simulink model "TV2016_CAN"  (Simulink 8.5)
settings: Solver=ode1  StartTime=0.0  StopTime=inf  FixedStep=0.001  RelTol=1e-3
PreLoadFcn:
  | FSE_Parameters
values from neighbouring files (symbols this model uses):
  car_params = Simulink_Car_params    [TV2016_parameters.m]
  i_Diff = 15.47    [TV2016_parameters.m]
  Kp = 1    [TV2016_parameters.m]
  settings = Simulink_Settings    [TV2016_parameters.m]
  SpdC_BCC = 0    [TV2016_parameters.m]
  Speed_Neg_sat = -21    [TV2016_parameters.m]
  Speed_Pos_sat = 21    [TV2016_parameters.m]
  Tn_n = 0    [TV2016_parameters.m]
  Use_Joystick = 1    [TV2016_parameters.m]
undefined symbols (not defined in the file or in its folder): canChannel
libraries: CarMaker4SL x139, simulink x18, canmsglib x10, simulink_extras x7, canlib x5, sldrtlib x1
(part 2 of 4)

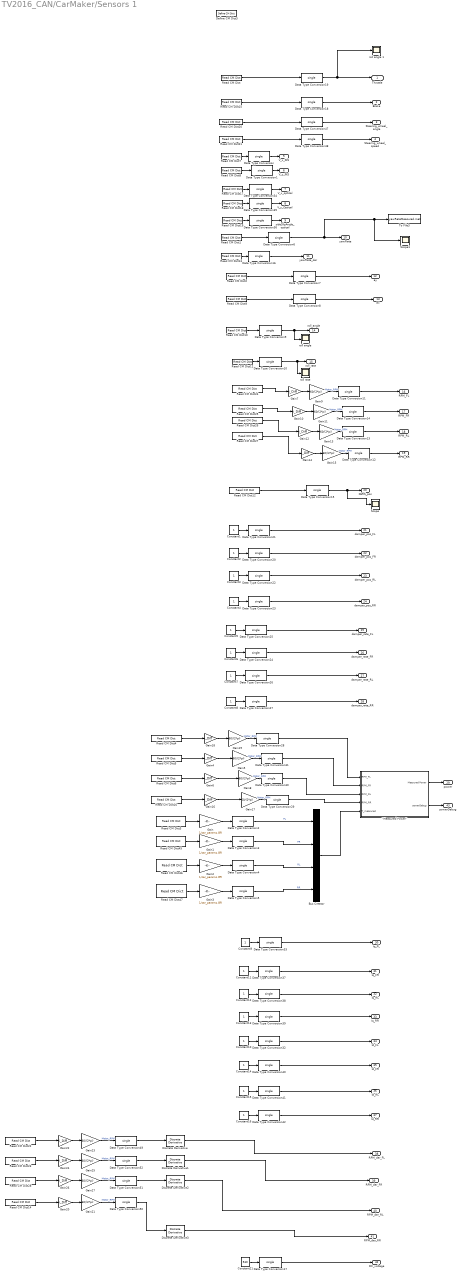
== system TV2016_CAN/CarMaker/Sensors 1 ==
  "\"Measured Power\"" : Subsystem
  Bus Creator : BusCreator  OutDataTypeStr=Bus: T_meas
      settings: InheritFromInputs=off
  Constant{1..16} (16 alike) : Constant
  Constant21 : Constant  Value=530
  Data Type Conversion{,1..42,47..52} (49 alike) : DataTypeConversion  OutDataTypeStr=single
  Define CM Dict3 : CarMaker4SL/Define CM Dict  xname=KERS_pos  xmono=off  xtype=Double  xdvaplace=None  xnstates=0  xfirststate=0  xinitial=0
  Discrete Derivative{,1..3} (4 alike) : simulink/Discrete/Discrete Derivative  gainval=1.0  ICPrevScaledInput=0.0  InputProcessing=Inherited  OutMin=[]  OutMax=[]  OutDataType=fixdt(1, 16)  OutScaling=2^-10  DoSatur=off
  Gain{,1..3} (4 alike) : Gain  Gain=1/car_params.GR
  Gain{4,6..7,10,12,14,16,18,20,22,24,26} (12 alike) : Gain  Gain=i_Diff
  Gain{5,8..9,11,13,15,17,19,21,23,25,27} (12 alike) : Gain  Gain=60/(2*pi)
  Read CM Dict : CarMaker4SL/Read CM Dict  xname=VC.Gas  xsync=off
  Read CM Dict1 : CarMaker4SL/Read CM Dict  xname=Vhcl.YawRate  xsync=off
  Read CM Dict10 : CarMaker4SL/Read CM Dict  xname=Vhcl.Roll  xsync=off
  Read CM Dict11 : CarMaker4SL/Read CM Dict  xname=Vhcl.RollVel  xsync=off
  Read CM Dict12 : CarMaker4SL/Read CM Dict  xname=KERS_pos  xsync=off
  Read CM Dict13 : CarMaker4SL/Read CM Dict  xname=Vhcl.YawAcc  xsync=off
  Read CM Dict14 : CarMaker4SL/Read CM Dict  xname=Car.WheelSpd_RR  xsync=off
  Read CM Dict15 : CarMaker4SL/Read CM Dict  xname=VC.Brake  xsync=off
  Read CM Dict16 : CarMaker4SL/Read CM Dict  xname=Car.WheelSpd_RR  xsync=off
  Read CM Dict17 : CarMaker4SL/Read CM Dict  xname=Car.vx  xsync=off
  Read CM Dict18 : CarMaker4SL/Read CM Dict  xname=Car.vy  xsync=off
  Read CM Dict19 : CarMaker4SL/Read CM Dict  xname=Car.SideSlipAngle  xsync=off
  Read CM Dict2 : CarMaker4SL/Read CM Dict  xname=Car.ay  xsync=off
  Read CM Dict20 : CarMaker4SL/Read CM Dict  xname=Vhcl.Steer.Ang  xsync=off
  Read CM Dict21 : CarMaker4SL/Read CM Dict  xname=Vhcl.Steer.Vel  xsync=off
  Read CM Dict22 : CarMaker4SL/Read CM Dict  xname=Car.WheelSpd_FL  xsync=off
  Read CM Dict23 : CarMaker4SL/Read CM Dict  xname=Car.WheelSpd_FR  xsync=off
  Read CM Dict24 : CarMaker4SL/Read CM Dict  xname=Car.WheelSpd_FL  xsync=off
  Read CM Dict25 : CarMaker4SL/Read CM Dict  xname=Car.WheelSpd_FR  xsync=off
  Read CM Dict26 : CarMaker4SL/Read CM Dict  xname=Car.WheelSpd_RL  xsync=off
  Read CM Dict27 : CarMaker4SL/Read CM Dict  xname=Car.WheelSpd_RR  xsync=off
  Read CM Dict28 : CarMaker4SL/Read CM Dict  xname=Car.WheelSpd_RL  xsync=off
  Read CM Dict3 : CarMaker4SL/Read CM Dict  xname=PT.WFL.Trq_Drive  xsync=off
  Read CM Dict4 : CarMaker4SL/Read CM Dict  xname=Car.WheelSpd_FL  xsync=off
  Read CM Dict45 : CarMaker4SL/Read CM Dict  xname=PT.WFR.Trq_Drive  xsync=off
  Read CM Dict46 : CarMaker4SL/Read CM Dict  xname=PT.WRL.Trq_Drive  xsync=off
  Read CM Dict47 : CarMaker4SL/Read CM Dict  xname=PT.WRR.Trq_Drive  xsync=off
  Read CM Dict5 : CarMaker4SL/Read CM Dict  xname=Car.WheelSpd_FR  xsync=off
  Read CM Dict6 : CarMaker4SL/Read CM Dict  xname=Car.WheelSpd_RL  xsync=off
  Read CM Dict7 : CarMaker4SL/Read CM Dict  xname=Car.vx  xsync=off
  Read CM Dict8 : CarMaker4SL/Read CM Dict  xname=Car.vy  xsync=off
  Read CM Dict9 : CarMaker4SL/Read CM Dict  xname=Car.ax  xsync=off
  Scope : Scope
      settings: SaveName=ScopeData77
  Scope1 : Scope
      settings: ShowLegends=on  TimeRange=2.184524711696869  YMin=-0.01  YMax=0.02  SaveName=ScopeData50
  To File3 : ToFile  Filename=yawRateMeasured.mat  MatrixName=rMeas  SaveFormat=Timeseries
  "roll angle " : Scope
      settings: ShowLegends=on  YMin=-17.5  YMax=17.5  SaveName=ScopeData63
  roll angle 1 : Scope
      settings: ShowLegends=on  YMin=-17.5  YMax=17.5  SaveName=ScopeData78
  roll rate : Scope
      settings: ShowLegends=on  YMin=-17.5  YMax=17.5  SaveName=ScopeData65
  "Throttle " : Outport
  "Brake " : Outport  Port=2
  "Steering_wheel_angle " : Outport  Port=3
  Steering_wheel_speed : Outport  Port=4
  V_x_INS : Outport  Port=5
  V_y_INS : Outport  Port=6
  V_x_optical : Outport  Port=7
  V_y_Optical : Outport  Port=8
  sideSlipAngle_optical : Outport  Port=9
  yawRate : Outport  Port=10
  yawRate_der : Outport  Port=11
  ay : Outport  Port=12
  "ax " : Outport  Port=13
  roll_angle : Outport  Port=14
  roll_rate : Outport  Port=15
  RPM_FL : Outport  Port=16
  RPM_FR : Outport  Port=17
  RPM_RL : Outport  Port=18
  RPM_RR : Outport  Port=19
  KERS_pos : Outport  Port=20
  damper_pos_FL : Outport  Port=21
  damper_pos_FR : Outport  Port=22
  damper_pos_RL : Outport  Port=23
  damper_pos_RR : Outport  Port=24
  damper_rate_FL : Outport  Port=25
  damper_rate_FR : Outport  Port=26
  damper_rate_RL : Outport  Port=27
  damper_rate_RR : Outport  Port=28
  power : Outport  Port=29
  Iq_FL : Outport  Port=30
  Iq_FR : Outport  Port=31
  Iq_RL : Outport  Port=32
  Iq_RR : Outport  Port=33
  Id_FL : Outport  Port=34
  Id_FR : Outport  Port=35
  Id_RL : Outport  Port=36
  Id_RR : Outport  Port=37
  RPM_der_FL : Outport  Port=38
  RPM_der_FR : Outport  Port=39
  RPM_der_RL : Outport  Port=40
  RPM_der_RR : Outport  Port=41
  DC_voltage : Outport  Port=42
  powerDebug : Outport  Port=43
  wires:
  Read CM Dict7/1 -> Data Type Conversion/1
  Read CM Dict8/1 -> Data Type Conversion1/1
  Read CM Dict1/1 -> Data Type Conversion6/1
  Data Type Conversion/1 -> V_x_INS/1
  Data Type Conversion1/1 -> V_y_INS/1
  Read CM Dict10/1 -> Data Type Conversion9/1
  Data Type Conversion9/1 -> "roll angle "/1, roll_angle/1
  Read CM Dict11/1 -> Data Type Conversion10/1
  Data Type Conversion10/1 -> roll rate/1, roll_rate/1
  Gain7/1 -> Gain9/1
  Read CM Dict24/1 -> Gain7/1
  Read CM Dict25/1 -> Gain10/1
  Gain10/1 -> Gain11/1
  Gain12/1 -> Gain13/1
  Gain14/1 -> Gain15/1
  Read CM Dict26/1 -> Gain12/1
  Read CM Dict27/1 -> Gain14/1
  Gain9/1 -> Data Type Conversion11/1  "Motor_RPM"
  Gain15/1 -> Data Type Conversion12/1  "Motor_RPM"
  Gain13/1 -> Data Type Conversion13/1  "Motor_RPM"
  Gain11/1 -> Data Type Conversion14/1  "Motor_RPM"
  Data Type Conversion11/1 -> RPM_FL/1
  Data Type Conversion14/1 -> RPM_FR/1
  Data Type Conversion13/1 -> RPM_RL/1
  Data Type Conversion12/1 -> RPM_RR/1
  Read CM Dict12/1 -> Data Type Conversion15/1
  Data Type Conversion15/1 -> Scope/1, KERS_pos/1
  Data Type Conversion7/1 -> ay/1
  Data Type Conversion8/1 -> "ax "/1
  Read CM Dict/1 -> Data Type Conversion19/1
  Read CM Dict15/1 -> Data Type Conversion18/1
  Data Type Conversion18/1 -> "Brake "/1
  Data Type Conversion19/1 -> roll angle 1/1, "Throttle "/1
  Data Type Conversion21/1 -> damper_pos_FL/1
  Constant1/1 -> Data Type Conversion21/1
  Data Type Conversion20/1 -> damper_pos_FR/1
  Constant2/1 -> Data Type Conversion20/1
  Data Type Conversion22/1 -> damper_pos_RL/1
  Constant3/1 -> Data Type Conversion22/1
  Data Type Conversion23/1 -> damper_pos_RR/1
  Constant4/1 -> Data Type Conversion23/1
  Data Type Conversion25/1 -> damper_rate_FL/1
  Constant5/1 -> Data Type Conversion25/1
  Data Type Conversion24/1 -> damper_rate_FR/1
  Constant6/1 -> Data Type Conversion24/1
  Data Type Conversion26/1 -> damper_rate_RL/1
  Constant7/1 -> Data Type Conversion26/1
  Data Type Conversion27/1 -> damper_rate_RR/1
  Constant8/1 -> Data Type Conversion27/1
  Read CM Dict3/1 -> Gain/1
  Read CM Dict45/1 -> Gain1/1
  Read CM Dict46/1 -> Gain2/1
  Read CM Dict47/1 -> Gain3/1
  Data Type Conversion2/1 -> Bus Creator/1  "FL"
  Data Type Conversion3/1 -> Bus Creator/2  "FR"
  Data Type Conversion4/1 -> Bus Creator/3  "RL"
  Data Type Conversion5/1 -> Bus Creator/4  "RR"
  Gain/1 -> Data Type Conversion2/1
  Gain1/1 -> Data Type Conversion3/1
  Gain2/1 -> Data Type Conversion4/1
  Gain3/1 -> Data Type Conversion5/1
  Bus Creator/1 -> "\"Measured Power\""/5(T_measured)
  Gain18/1 -> Gain19/1
  Read CM Dict4/1 -> Gain18/1
  Read CM Dict5/1 -> Gain4/1
  Gain4/1 -> Gain5/1
  Gain6/1 -> Gain8/1
  Gain16/1 -> Gain17/1
  Read CM Dict6/1 -> Gain6/1
  Read CM Dict16/1 -> Gain16/1
  Gain19/1 -> Data Type Conversion28/1  "Motor_RPM"
  Gain17/1 -> Data Type Conversion29/1  "Motor_RPM"
  Gain8/1 -> Data Type Conversion30/1  "Motor_RPM"
  Gain5/1 -> Data Type Conversion31/1  "Motor_RPM"
  Data Type Conversion29/1 -> "\"Measured Power\""/4(RPM_RR)
  Data Type Conversion30/1 -> "\"Measured Power\""/3(RPM_RL)
  Data Type Conversion31/1 -> "\"Measured Power\""/2(RPM_FR)
  Data Type Conversion28/1 -> "\"Measured Power\""/1(RPM_FL)
  "\"Measured Power\""/1("Measured Power ") -> power/1
  "\"Measured Power\""/2(powerDebug) -> powerDebug/1
  Data Type Conversion33/1 -> Iq_FL/1
  Constant9/1 -> Data Type Conversion33/1
  Data Type Conversion32/1 -> Id_FL/1
  Constant10/1 -> Data Type Conversion32/1
  Read CM Dict9/1 -> Data Type Conversion8/1
  Read CM Dict2/1 -> Data Type Conversion7/1
  Read CM Dict17/1 -> Data Type Conversion34/1
  Read CM Dict18/1 -> Data Type Conversion35/1
  Data Type Conversion34/1 -> V_x_optical/1
  Data Type Conversion35/1 -> V_y_Optical/1
  Data Type Conversion36/1 -> sideSlipAngle_optical/1
  Read CM Dict19/1 -> Data Type Conversion36/1
  Data Type Conversion37/1 -> Iq_FR/1
  Constant11/1 -> Data Type Conversion37/1
  Data Type Conversion38/1 -> Iq_RL/1
  Constant12/1 -> Data Type Conversion38/1
  Data Type Conversion39/1 -> Iq_RR/1
  Constant13/1 -> Data Type Conversion39/1
  Data Type Conversion40/1 -> Id_FR/1
  Constant14/1 -> Data Type Conversion40/1
  Data Type Conversion41/1 -> Id_RL/1
  Constant15/1 -> Data Type Conversion41/1
  Data Type Conversion42/1 -> Id_RR/1
  Constant16/1 -> Data Type Conversion42/1
  Read CM Dict20/1 -> Data Type Conversion47/1
  Read CM Dict21/1 -> Data Type Conversion48/1
  Data Type Conversion47/1 -> "Steering_wheel_angle "/1
  Data Type Conversion48/1 -> Steering_wheel_speed/1
  Data Type Conversion16/1 -> yawRate_der/1
  Read CM Dict13/1 -> Data Type Conversion16/1
  Data Type Conversion17/1 -> DC_voltage/1
  Constant21/1 -> Data Type Conversion17/1
  Gain22/1 -> Gain23/1
  Read CM Dict22/1 -> Gain22/1
  Read CM Dict23/1 -> Gain24/1
  Gain24/1 -> Gain25/1
  Gain26/1 -> Gain27/1
  Gain20/1 -> Gain21/1
  Read CM Dict28/1 -> Gain26/1
  Read CM Dict14/1 -> Gain20/1
  Gain23/1 -> Data Type Conversion49/1  "Motor_RPM"
  Gain21/1 -> Data Type Conversion50/1  "Motor_RPM"
  Gain27/1 -> Data Type Conversion51/1  "Motor_RPM"
  Gain25/1 -> Data Type Conversion52/1  "Motor_RPM"
  Data Type Conversion50/1 -> Discrete Derivative3/1
  Data Type Conversion51/1 -> Discrete Derivative2/1
  Data Type Conversion52/1 -> Discrete Derivative1/1
  Data Type Conversion49/1 -> Discrete Derivative/1
  Discrete Derivative/1 -> RPM_der_FL/1
  Discrete Derivative1/1 -> RPM_der_FR/1
  Discrete Derivative2/1 -> RPM_der_RL/1
  Discrete Derivative3/1 -> RPM_der_RR/1
  Data Type Conversion6/1 -> To File3/1, Scope1/1, yawRate/1

== system TV2016_CAN/CarMaker/VehicleControl1 ==
  note: <Your model here>
  note: When implementing a vehicle control model,
      | be sure to add '-disablevehiclecontrol' to the command line arguments
      | in the CarMaker Model Configuration block.
      | Otherwise your model will possibly not see the original DrivMan signals
      | on its inputs, but those of a currently activated C-coded vehicle control model instead.
  Sync_In : Inport
  DrivMan.In : Inport  Port=2
  Bus Creator2 : BusCreator  Inputs=2
  CreateBus Vhcl.Misc : Subsystem
  CreateBus Vhcl.Wheel.In : Subsystem
  CreateBus VhclCtrl : Subsystem
  CreateBus VhclCtrl.PT : Subsystem
  CreateBus VhclCtrl.Steering : Subsystem
  Demux2 : Demux  Outputs=2
  VehicleControl : S-Function  FunctionName=CM_Sfun  Parameters='VehicleControl'
  VehicleControlUpd : S-Function  FunctionName=CM_Sfun  Parameters='VehicleControlUpd'
  Sync_Out : Outport
  Vhcl.Model.Source : Outport  Port=2
  VhclCtrl.Steering : Outport  Port=3
  Vhcl.Wheel.In : Outport  Port=4
  Vhcl.Misc : Outport  Port=5
  VhclCtrl.Brake : Outport  Port=6
  VhclCtrl.PT : Outport  Port=7
  wires:
  CreateBus VhclCtrl/1(Out) -> VehicleControlUpd/2
  VehicleControl/2 -> CreateBus VhclCtrl/1(In)
  VehicleControlUpd/2 -> Vhcl.Model.Source/1
  VehicleControlUpd/4 -> CreateBus Vhcl.Wheel.In/1(In1)
  VehicleControlUpd/5 -> CreateBus Vhcl.Misc/1(In1)
  VehicleControlUpd/6 -> Demux2/1
  VehicleControlUpd/7 -> CreateBus VhclCtrl.PT/1(In1)
  VehicleControlUpd/3 -> CreateBus VhclCtrl.Steering/1(In1)
  CreateBus Vhcl.Misc/1(Out1) -> Vhcl.Misc/1
  CreateBus Vhcl.Wheel.In/1(Out1) -> Vhcl.Wheel.In/1
  DrivMan.In/1 -> VehicleControl/2
  VehicleControl/1 -> VehicleControlUpd/1
  Sync_In/1 -> VehicleControl/1
  CreateBus VhclCtrl.PT/1(Out1) -> VhclCtrl.PT/1
  Bus Creator2/1 -> VhclCtrl.Brake/1
  CreateBus VhclCtrl.Steering/1(Out1) -> VhclCtrl.Steering/1
  VehicleControlUpd/1 -> Sync_Out/1
  Demux2/2 -> Bus Creator2/2  "VhclCtrl BrakePark"
  Demux2/1 -> Bus Creator2/1  "VhclCtrl Brake"

== system TV2016_CAN/CarMaker/Debug Information /Motor Rpm log   ==
  Abs : Abs
  Discrete Derivative : simulink/Discrete/Discrete Derivative  gainval=1.0  ICPrevScaledInput=0.0  InputProcessing=Inherited  OutMin=[]  OutMax=[]  OutDataType=fixdt(1, 16)  OutScaling=2^-10  DoSatur=off
  Fl_derivate : Scope
      settings: ShowLegends=on  TimeRange=3.722  YMin=0  YMax=10000  SaveName=ScopeData57
  Gain{7,10,12,14} (4 alike) : Gain  Gain=i_Diff
  Gain{9,11,13,15} (4 alike) : Gain  Gain=60/(2*pi)
  Mux1 : Mux
  Rate Transition : RateTransition  OutPortSampleTime=settings.control_system_sample_time
  Read CM Dict24 : CarMaker4SL/Read CM Dict  xname=Car.WheelSpd_FL  xsync=off
  Read CM Dict25 : CarMaker4SL/Read CM Dict  xname=Car.WheelSpd_FR  xsync=off
  Read CM Dict26 : CarMaker4SL/Read CM Dict  xname=Car.WheelSpd_RL  xsync=off
  Read CM Dict27 : CarMaker4SL/Read CM Dict  xname=Car.WheelSpd_RR  xsync=off
  Saturation : Saturate  UpperLimit=50000
  To File : ToFile  Filename=MotorRPMS.mat  MatrixName=MotorRpms  SaveFormat=Timeseries
  eng rot : Scope
      settings: ShowLegends=on  TimeRange=1.853487603305785  YMin=11642.1568627451  YMax=19093.13725490196  SaveName=ScopeData55
  wires:
  Gain7/1 -> Gain9/1
  Gain9/1 -> Mux1/1, Rate Transition/1  "Motor_RPM"
  Read CM Dict24/1 -> Gain7/1
  Read CM Dict25/1 -> Gain10/1
  Gain10/1 -> Gain11/1
  Gain11/1 -> Mux1/2  "Motor_RPM"
  Gain12/1 -> Gain13/1
  Gain13/1 -> Mux1/3  "Motor_RPM"
  Gain14/1 -> Gain15/1
  Gain15/1 -> Mux1/4  "Motor_RPM"
  Read CM Dict26/1 -> Gain12/1
  Read CM Dict27/1 -> Gain14/1
  Mux1/1 -> eng rot/1, To File/1
  Discrete Derivative/1 -> Abs/1
  Abs/1 -> Saturation/1
  Saturation/1 -> Fl_derivate/1
  Rate Transition/1 -> Discrete Derivative/1

== system TV2016_CAN/CarMaker/IPG Vehicle1/Brake ==
  note: <Your model here>
  note: When replacing the entire braking system,
      | be sure to add '-disablebrake' to the command line arguments
      | in the CarMaker Model Configuration block.
  Sync_In : Inport
  Brake.IF.In : Inport  Port=2
  VhclCtrl.Brake : Inport  Port=3
  Brake : S-Function  FunctionName=CM_Sfun  Parameters='Brake'
  BrakeUpd : S-Function  FunctionName=CM_Sfun  Parameters='BrakeUpd'
  BusCreator : BusCreator  Inputs=12
  CreateBus Vhcl.Wheel.PT : Subsystem
  Demux : Demux  Outputs=12
  Sync_Out : Outport
  Vhcl.Wheel.PT : Outport  Port=2
  wires:
  BrakeUpd/1 -> Sync_Out/1
  Brake/1 -> BrakeUpd/1  "Sync"
  Brake.IF.In/1 -> Brake/2
  VhclCtrl.Brake/1 -> Brake/3
  Brake/2 -> Demux/1
  BusCreator/1 -> BrakeUpd/2
  Sync_In/1 -> Brake/1
  Demux/12 -> BusCreator/12  "Brake IF Trq_Reg_trg RR"
  Demux/11 -> BusCreator/11  "Brake IF Trq_Reg_trg RL"
  Demux/10 -> BusCreator/10  "Brake IF Trq_Reg_trg FR"
  Demux/9 -> BusCreator/9  "Brake IF Trq_Reg_trg FL"
  Demux/8 -> BusCreator/8  "Brake IF Trq_PB RR"
  Demux/7 -> BusCreator/7  "Brake IF Trq_PB RL"
  Demux/6 -> BusCreator/6  "Brake IF Trq_PB FR"
  Demux/5 -> BusCreator/5  "Brake IF Trq_PB FL"
  Demux/4 -> BusCreator/4  "Brake IF Trq_WB RR"
  Demux/3 -> BusCreator/3  "Brake IF Trq_WB RL"
  Demux/2 -> BusCreator/2  "Brake IF Trq_WB FR"
  Demux/1 -> BusCreator/1  "Brake IF Trq_WB FL"
  BrakeUpd/2 -> CreateBus Vhcl.Wheel.PT/1(In)
  CreateBus Vhcl.Wheel.PT/1(Out) -> Vhcl.Wheel.PT/1

== system TV2016_CAN/CarMaker/IPG Vehicle1/CarAndTrailer ==
  Sync_In : Inport
  VhclCtrl.Steering : Inport  Port=2
  Vhcl.Wheel.In : Inport  Port=3
  Vhcl.Misc : Inport  Port=4
  CarAndTrailerUpd : Subsystem
  Forces : Subsystem
  Ground : Ground
  Kinematics : Subsystem
  Kinetics : Subsystem
  Steering : Subsystem
  Terminator : Terminator
  Terminator1 : Terminator
  Trailer : Subsystem
  Sync_Out : Outport
  Brake.IF.In : Outport  Port=2
  wires:
  Trailer/9(Car.Hitch.FrcTrq) -> CarAndTrailerUpd/9(Car.Hitch.FrcTrq)
  Trailer/8(Vhcl.Wheel.RR) -> CarAndTrailerUpd/8(Vhcl.Wheel.RR)
  Trailer/7(Vhcl.Wheel.RL) -> CarAndTrailerUpd/7(Vhcl.Wheel.RL)
  Trailer/6(Vhcl.Wheel.FR) -> CarAndTrailerUpd/6(Vhcl.Wheel.FR)
  Trailer/5(Vhcl.Wheel.FL) -> CarAndTrailerUpd/5(Vhcl.Wheel.FL)
  Trailer/4(Vhcl.PoI) -> CarAndTrailerUpd/4(Vhcl.PoI)
  Trailer/3(Vhcl.Motion) -> CarAndTrailerUpd/3(Vhcl.Motion)
  Trailer/2(Vhcl.Steering) -> CarAndTrailerUpd/2(Vhcl.Steering)
  Trailer/1(Sync_Out) -> CarAndTrailerUpd/1(Sync_In)
  CarAndTrailerUpd/2(Brake.IF.In) -> Brake.IF.In/1
  CarAndTrailerUpd/1(Sync_Out) -> Sync_Out/1
  Vhcl.Misc/1 -> Terminator1/1
  Vhcl.Wheel.In/1 -> Terminator/1
  Kinetics/6(WheelCarrier.Misc) -> Trailer/6(WheelCarrier.Misc)
  Kinetics/5(Car.Trq_T2W) -> Trailer/5(Car.Trq_T2W)
  Steering/2(Steer.IF) -> Kinematics/2(Steer.IF)
  Kinetics/4(Car.Fr1) -> Trailer/4(Car.Fr1)
  Kinetics/3(Car.Hitch) -> Trailer/3(Car.Hitch)
  Kinetics/2(Trailer.Load) -> Trailer/2(Trailer.Load)
  VhclCtrl.Steering/1 -> Steering/2(VhclCtrl.Steering)
  Sync_In/1 -> Steering/1(Sync_In)
  Steering/1(Sync_Out) -> Kinematics/1(Sync_In)
  Kinetics/1(Sync_Out) -> Trailer/1(Sync_In)
  Ground/1 -> CarAndTrailerUpd/10(Vhcl.Fr1A)
  Forces/11(FStabi) -> Kinetics/11(FStabi)
  Forces/10(FDamp) -> Kinetics/10(FDamp)
  Forces/9(FSpring) -> Kinetics/9(FSpring)
  Forces/8(TireRR_Out) -> Kinetics/8(TireRR.Out)
  Forces/7(TireRL_Out) -> Kinetics/7(TireRL.Out)
  Forces/6(TireFR_Out) -> Kinetics/6(TireFR.Out)
  Forces/5(TireFL_Out) -> Kinetics/5(TireFL.Out)
  Forces/4(Car.Load) -> Kinetics/4(Car.Load)
  Forces/2(Car.Virtual) -> Kinetics/2(Car.Virtual)
  Kinematics/6(lSpring) -> Forces/6(lSpring)
  Kinematics/7(vDamp) -> Forces/7(vDamp)
  Forces/3(Car.Aero) -> Kinetics/3(Car.Aero)
  Forces/1(Sync_Out) -> Kinetics/1(Sync_In)
  Kinematics/5(TireRR_In) -> Forces/5(TireRR_In)
  Kinematics/4(TireRL_In) -> Forces/4(TireRL_In)
  Kinematics/3(TireFR_In) -> Forces/3(TireFR_In)
  Kinematics/2(TireFL_In) -> Forces/2(TireFL_In)
  Kinematics/1(Sync_Out) -> Forces/1(Sync_In)
  Kinematics/8(lStabi) -> Forces/8(lStabi)
  Forces/12(FBuf) -> Kinetics/12(FBuf)
  Kinematics/9(lBuf) -> Forces/9(lBuf)

== system TV2016_CAN/CarMaker/IPG Vehicle1/PowerTrain ==
  note: When replacing the entire powertrain,
      | be sure to add '-disablepowertrain' to the command line arguments
      | in the CarMaker Model Configuration block.
  Sync_In : Inport
  Vhcl.Wheel.PT : Inport  Port=2
  VhclCtrl.PT : Inport  Port=3
  BusCreator : BusCreator  Inputs=40
  Demux : Demux  Outputs=40
  Electric Powertrain : Subsystem
  PowerTrain : S-Function  FunctionName=CM_Sfun  Parameters='PowerTrain'
  PowerTrainUpd : S-Function  FunctionName=CM_Sfun  Parameters='PowerTrainUpd'
  Terminator{1..6} (6 alike) : Terminator
  Sync_Out : Outport
  wires:
  Sync_In/1 -> PowerTrain/1
  PowerTrain/2 -> Demux/1
  PowerTrainUpd/1 -> Sync_Out/1
  PowerTrain/1 -> PowerTrainUpd/1  "Sync"
  Demux/1 -> BusCreator/1  "PT IF Ignition"
  Demux/2 -> Terminator2/1  "PT IF OperationState"
  Demux/4 -> ?  "PT IF GearNo"
  Demux/5 -> Terminator1/1  "PT IF Engine_rotv"
  Demux/7 -> ?  "PT IF Trq_Supp2Bdy1 x"
  Demux/8 -> ?  "PT IF Trq_Supp2Bdy1 y"
  Demux/9 -> ?  "PT IF Trq_Supp2Bdy1 z"
  Demux/10 -> ?  "PT IF Trq_Supp2BdyEng x"
  Demux/11 -> ?  "PT IF Trq_Supp2BdyEng y"
  Demux/12 -> ?  "PT IF DL_iDiff_mean"
  Demux/13 -> BusCreator/13  "PT IF WFL rot"
  Demux/14 -> BusCreator/14  "PT IF WFL rotv"
  Demux/15 -> ?  "PT IF WFL Trq_B2W"
  Demux/16 -> Terminator6/1  "PT IF WFL Trq_Drive"
  Demux/17 -> ?  "PT IF WFL Trq_Supp2WC"
  Demux/18 -> ?  "PT IF WFL Trq_BrakeReg"
  Demux/19 -> ?  "PT IF WFL Trq_BrakeReg_max"
  Demux/20 -> BusCreator/20  "PT IF WFR rot"
  Demux/21 -> BusCreator/21  "PT IF WFR rotv"
  Demux/22 -> ?  "PT IF WFR Trq_B2W"
  Demux/23 -> Terminator5/1  "PT IF WFR Trq_Drive"
  Demux/24 -> ?  "PT IF WFR Trq_Supp2WC"
  Demux/25 -> ?  "PT IF WFR Trq_BrakeReg"
  Demux/26 -> ?  "PT IF WFR Trq_BrakeReg_max"
  Demux/27 -> BusCreator/27  "PT IF WRL rot"
  Demux/28 -> BusCreator/28  "PT IF WRL rotv"
  Demux/29 -> ?  "PT IF WRL Trq_B2W"
  Demux/30 -> Terminator4/1  "PT IF WRL Trq_Drive"
  Demux/31 -> ?  "PT IF WRL Trq_Supp2WC"
  Demux/32 -> ?  "PT IF WRL Trq_BrakeReg"
  Demux/33 -> ?  "PT IF WRL Trq_BrakeReg_max"
  Demux/34 -> BusCreator/34  "PT IF WRR rot"
  Demux/35 -> BusCreator/35  "PT IF WRR rotv"
  Demux/36 -> ?  "PT IF WRR Trq_B2W"
  Demux/37 -> Terminator3/1  "PT IF WRR Trq_Drive"
  Demux/38 -> ?  "PT IF WRR Trq_Supp2WC"
  Demux/39 -> ?  "PT IF WRR Trq_BrakeReg"
  Demux/40 -> ?  "PT IF WRR Trq_BrakeReg_max"
  VhclCtrl.PT/1 -> PowerTrain/3
  Vhcl.Wheel.PT/1 -> PowerTrain/2
  BusCreator/1 -> PowerTrainUpd/2
  Electric Powertrain/2(PT.Engine.rotv) -> ?
  Demux/6 -> ?  "PT IF Engine_Trq (EngineControl)"
  Demux/3 -> BusCreator/3  "PT IF OperationError"
  Electric Powertrain/1(PT.OperationState) -> BusCreator/2
  Electric Powertrain/3(T_FL) -> BusCreator/16
  Electric Powertrain/4(T_FR) -> BusCreator/23
  Electric Powertrain/5(T_RL) -> BusCreator/30
  Electric Powertrain/6(T_RR) -> BusCreator/37

== system TV2016_CAN/CarMaker/Sensors 1/"Measured Power" ==
  RPM_FL : Inport
  RPM_FR : Inport  Port=2
  RPM_RL : Inport  Port=3
  RPM_RR : Inport  Port=4
  T_measured : Inport  Port=5
  2-D Lookup Table{,1..3} (4 alike) : Lookup_n-D  BreakpointsForDimension1=single([1.3,2.7,5.4,7.9,10.4,12.5,14.4,16.0,17.4,18.5,19.6]);  BreakpointsForDimension2=single([500,1000,2000,3000,4000,6000,10000,12000,15000,19000]);  Table=single(reshape([0.6437000036239624,0.5799999833106995,0.44999998807907104,0.3499999940395355,0.28999999165534973,0.23999999463558197,0.20000000298023224,0.17000000178813934,0.14000000059604645,0.12999999523162842,0.10999999940395355,0.7099999785423279,0.699999988079071,0.6100000143051148,0.5099999904632568,0.4399999976158142,0.3799999952316284,0.33000001311302185,0.28999999165534973,0.25,0.2199999988079071,0.20000000298023224,0.7300000190734863,0.7699999809265137,0.7300000190734863,0.6700000166893005,0.6100000143051148,0.550000011920929,0.5,0.44999998807907104,0.4000000059604645,0.36000001430511475,0.33000001311302185,0.7400000095367432,0.800000011920929,0.7900000214576721,0.7400000095367432,0.6899999976158142,0.6399999856948853,0.5899999737739563,0.5400000214576721,0.5,0.46000000834465027,0.41999998688697815,0.75,0.8199999928474426,0.8199999928474426,0.7799999713897705,0.7400000095367432,0.699999988079071,0.6600000262260437,0.6100000143051148,0.5699999928474426,0.5299999713897705,0.49000000953674316,0.7599999904632568,0.8399999737739563,0.8500000238418579,0.8299999833106995,0.800000011920929,0.7699999809265137,0.7400000095367432,0.699999988079071,0.6600000262260437,0.6200000047683716,0.5899999737739563,0.7699999809265137,0.8500000238418579,0.8799999952316284,0.8700000047683716,0.8600000143051148,0.8399999737739563,0.8100000023841858,0.7799999713897705,0.7599999904632568,0.7200000286102295,0.699999988079071,0.7699999809265137,0.8500000238418579,0.8899999856948853,0.8799999952316284,0.8700000047683716,0.8500000238418579,0.8299999833106995,0.8100000023841858,0.7799999713897705,0.7599999904632568,0.7300000190734863,0.7699999809265137,0.8600000143051148,0.8999999761581421,0.8999999761581421,0.8899999856948853,0.8700000047683716,0.8500000238418579,0.8299999833106995,0.8100000023841858,0.7900000214576721,0.6700000166893005,0.7799999713897705,0.8600000143051148,0.8999999761581421,0.9100000262260437,0.8999999761581421,0.8899999856948853,0.8700000047683716,0.8600000143051148,0.8299999833106995,0.7699999809265137,0.699999988079071],11,10));  ExtrapMethod=Clip  UseLastTableValue=on  InternalRulePriority=Speed  RndMeth=Simplest  InputSameDT=on
  Abs{,1..3} (4 alike) : Abs
  Add : Sum  Inputs=++++
  Bus Creator : BusCreator  Inputs=8  OutDataTypeStr=Bus: PowerDebug
      settings: InheritFromInputs=off
  Divide{,1..3} (4 alike) : Product  Inputs=*/
  MATLAB Function : MATLAB Function  TreatAsAtomicUnit=on
  Product{,1..3} (4 alike) : Product
  Switch{,1..3} (4 alike) : Switch  Criteria=u2 > Threshold
  fsact1 : Scope
      settings: ShowLegends=on  TimeRange=10  YMin=0  YMax=14  SaveName=ScopeData35
  "Measured Power " : Outport
  powerDebug : Outport  Port=2
  wires:
  MATLAB Function/2(T_FL) -> Abs/1
  MATLAB Function/3(RPM_FL) -> 2-D Lookup Table/2
  MATLAB Function/5(T_FR) -> Abs1/1
  MATLAB Function/8(T_RL) -> Abs2/1
  MATLAB Function/11(T_RR) -> Abs3/1
  MATLAB Function/12(RPM_RR) -> 2-D Lookup Table3/2
  Abs/1 -> 2-D Lookup Table/1
  Abs1/1 -> fsact1/1, 2-D Lookup Table1/1
  Abs2/1 -> 2-D Lookup Table2/1
  Abs3/1 -> 2-D Lookup Table3/1
  2-D Lookup Table/1 -> Divide/2, Product/2
  MATLAB Function/1(Pm_FL) -> Product/1, Switch/2, Divide/1, Bus Creator/1
  Add/1 -> "Measured Power "/1
  2-D Lookup Table1/1 -> Divide1/2, Product1/2
  2-D Lookup Table2/1 -> Divide2/2, Product2/2
  2-D Lookup Table3/1 -> Product3/2, Divide3/2
  MATLAB Function/7(Pm_RL) -> Bus Creator/5, Switch2/2, Product2/1, Divide2/1
  MATLAB Function/10(Pm_RR) -> Bus Creator/7, Switch3/2, Product3/1, Divide3/1
  Bus Creator/1 -> powerDebug/1
  T_measured/1 -> MATLAB Function/5(T)
  MATLAB Function/6(RPM_FR) -> 2-D Lookup Table1/2
  MATLAB Function/9(RPM_RL) -> 2-D Lookup Table2/2
  RPM_FL/1 -> MATLAB Function/1(RPM_FL_IN)
  RPM_FR/1 -> MATLAB Function/2(RPM_FR_IN)
  RPM_RL/1 -> MATLAB Function/3(RPM_RL_IN)
  RPM_RR/1 -> MATLAB Function/4(RPM_RR_IN)
  Divide/1 -> Switch/1
  Product/1 -> Switch/3
  MATLAB Function/4(Pm_FR) -> Bus Creator/3, Product1/1, Switch1/2, Divide1/1
  Divide1/1 -> Switch1/1
  Product1/1 -> Switch1/3
  Divide2/1 -> Switch2/1
  Product2/1 -> Switch2/3
  Divide3/1 -> Switch3/1
  Product3/1 -> Switch3/3
  Switch1/1 -> Bus Creator/4, Add/2  "Pe_FR"
  Switch3/1 -> Add/4, Bus Creator/8  "Pe_RR"
  Switch2/1 -> Bus Creator/6, Add/3  "Pe_RL"
  Switch/1 -> Bus Creator/2, Add/1  "Pe_FL"

== system TV2016_CAN/CarMaker/VehicleControl1/CreateBus Vhcl.Misc ==
  In1 : Inport
  Bus Creator5 : BusCreator  Inputs=11
  Demux5 : Demux  Outputs=11
  Out1 : Outport
  wires:
  Demux5/11 -> Bus Creator5/11  "Vhcl Wind_vel_0 z"
  Demux5/10 -> Bus Creator5/10  "Vhcl Wind_vel_0 y"
  Demux5/9 -> Bus Creator5/9  "Vhcl Wind_vel_0 x"
  Demux5/8 -> Bus Creator5/8  "Vhcl DL2BdyEng y"
  Demux5/7 -> Bus Creator5/7  "Vhcl DL2BdyEng x"
  Demux5/6 -> Bus Creator5/6  "Vhcl TrqDL2Bdy1B z"
  Demux5/5 -> Bus Creator5/5  "Vhcl TrqDL2Bdy1B y"
  Demux5/4 -> Bus Creator5/4  "Vhcl TrqDL2Bdy1B x"
  Demux5/3 -> Bus Creator5/3  "Vhcl Trq_DL2Bdy1 z"
  In1/1 -> Demux5/1
  Bus Creator5/1 -> Out1/1
  Demux5/2 -> Bus Creator5/2  "Vhcl Trq_DL2Bdy1 y"
  Demux5/1 -> Bus Creator5/1  "Vhcl Trq_DL2Bdy1 x"

== system TV2016_CAN/CarMaker/VehicleControl1/CreateBus Vhcl.Wheel.In ==
  In1 : Inport
  Bus Creator1 : BusCreator  Inputs=12
  Demux1 : Demux  Outputs=12
  Out1 : Outport
  wires:
  Demux1/12 -> Bus Creator1/12  "Vhcl Wheel RR rotv"
  Demux1/11 -> Bus Creator1/11  "Vhcl Wheel RR Trq_DL2WC"
  Demux1/10 -> Bus Creator1/10  "Vhcl Wheel RR Trq_B2WC"
  Demux1/9 -> Bus Creator1/9  "Vhcl Wheel RL rotv"
  Demux1/8 -> Bus Creator1/8  "Vhcl Wheel RL Trq_DL2WC"
  Demux1/7 -> Bus Creator1/7  "Vhcl Wheel RL Trq_B2WC"
  Demux1/6 -> Bus Creator1/6  "Vhcl Wheel FR rotv"
  Demux1/5 -> Bus Creator1/5  "Vhcl Wheel FR Trq_DL2WC"
  Demux1/4 -> Bus Creator1/4  "Vhcl Wheel FR Trq_B2WC"
  Demux1/3 -> Bus Creator1/3  "Vhcl Wheel FL rotv"
  In1/1 -> Demux1/1
  Bus Creator1/1 -> Out1/1
  Demux1/2 -> Bus Creator1/2  "Vhcl Wheel FL Trq_DL2WC"
  Demux1/1 -> Bus Creator1/1  "Vhcl Wheel FL Trq_B2WC"

== system TV2016_CAN/CarMaker/VehicleControl1/CreateBus VhclCtrl ==
  In : Inport
  Add KERS : MATLAB Function  TreatAsAtomicUnit=on
  BusCreator : BusCreator  Inputs=29
  Constant : Constant  Value=Use_Joystick
  Constant1 : Constant  Value=Use_Joystick
  Constant2 : Constant  Value=Use_Joystick
  Data Type Conversion : DataTypeConversion  OutDataTypeStr=double
  Demux : Demux  Outputs=29
  RacingwheelInterface : Subsystem
  Switch : Switch  Criteria=u2 > Threshold
  Switch1 : Switch  Criteria=u2 > Threshold
  Switch2 : Switch  Criteria=u2 > Threshold
  Write CM Dict1 : CarMaker4SL/Write CM Dict  xname=KERS_pos  xsync=off
  Out : Outport
  wires:
  In/1 -> Demux/1
  BusCreator/1 -> Out/1
  Demux/1 -> BusCreator/1  "VhclCtrl SST"
  Demux/2 -> BusCreator/2  "VhclCtrl Key"
  Demux/3 -> BusCreator/3  "VhclCtrl UserSignal0"
  Demux/4 -> BusCreator/4  "VhclCtrl UserSignal1"
  Demux/5 -> BusCreator/5  "VhclCtrl UserSignal2"
  Demux/6 -> BusCreator/6  "VhclCtrl UserSignal3"
  Demux/7 -> BusCreator/7  "VhclCtrl UserSignal4"
  Demux/8 -> BusCreator/8  "VhclCtrl GearNo"
  Demux/9 -> BusCreator/9  "VhclCtrl SelectorCtrl"
  Demux/10 -> Add KERS/1(brake_pedal)  "VhclCtrl Brake"
  Demux/11 -> BusCreator/11  "VhclCtrl BrakePark"
  Demux/12 -> BusCreator/12  "VhclCtrl Clutch"
  Demux/13 -> Switch1/1  "VhclCtrl Gas"
  Demux/14 -> Switch/1  "VhclCtrl Steering Ang"
  Demux/15 -> BusCreator/15  "VhclCtrl Steering AngVel"
  Demux/16 -> BusCreator/16  "VhclCtrl Steering AngAcc"
  Demux/17 -> BusCreator/17  "VhclCtrl Steering Trq"
  Demux/18 -> BusCreator/18  "VhclCtrl Lights LowBeam"
  Demux/19 -> BusCreator/19  "VhclCtrl Lights HighBeam"
  Demux/20 -> BusCreator/20  "VhclCtrl Lights Daytime"
  Demux/21 -> BusCreator/21  "VhclCtrl Lights ParkL"
  Demux/22 -> BusCreator/22  "VhclCtrl Lights ParkR"
  Demux/23 -> BusCreator/23  "VhclCtrl Lights IndL"
  Demux/24 -> BusCreator/24  "VhclCtrl Lights IndR"
  Demux/25 -> BusCreator/25  "VhclCtrl Lights FogFrontL"
  Demux/26 -> BusCreator/26  "VhclCtrl Lights FogFrontR"
  Demux/27 -> BusCreator/27  "VhclCtrl Lights FogRear"
  Demux/28 -> BusCreator/28  "VhclCtrl Lights Brake"
  Demux/29 -> BusCreator/29  "VhclCtrl Lights Reverse"
  RacingwheelInterface/1("Steering ") -> Switch/3
  RacingwheelInterface/2(throttleinoput) -> Switch1/3
  Constant/1 -> Switch/2
  Constant1/1 -> Switch1/2
  Constant2/1 -> Switch2/2
  RacingwheelInterface/3(brake input) -> Switch2/3
  Switch/1 -> BusCreator/14
  Switch1/1 -> BusCreator/13
  Switch2/1 -> BusCreator/10
  Add KERS/1(KERS_pos) -> Data Type Conversion/1
  Data Type Conversion/1 -> Write CM Dict1/1
  Add KERS/2(brake_pos) -> Switch2/1

== system TV2016_CAN/CarMaker/VehicleControl1/CreateBus VhclCtrl.PT ==
  In1 : Inport
  BusCreator : BusCreator  Inputs=11
  Demux : Demux  Outputs=11
  Out1 : Outport
  wires:
  In1/1 -> Demux/1
  BusCreator/1 -> Out1/1
  Demux/1 -> BusCreator/1  "VhclCtrl SST"
  Demux/2 -> BusCreator/2  "VhclCtrl Key"
  Demux/3 -> BusCreator/3  "VhclCtrl UserSignal0"
  Demux/4 -> BusCreator/4  "VhclCtrl UserSignal1"
  Demux/5 -> BusCreator/5  "VhclCtrl UserSignal2"
  Demux/6 -> BusCreator/6  "VhclCtrl UserSignal3"
  Demux/7 -> BusCreator/7  "VhclCtrl UserSignal4"
  Demux/8 -> BusCreator/8  "VhclCtrl GearNo"
  Demux/9 -> BusCreator/9  "VhclCtrl SelectorCtrl"
  Demux/10 -> BusCreator/10  "VhclCtrl Clutch"
  Demux/11 -> BusCreator/11  "VhclCtrl Gas"

== system TV2016_CAN/CarMaker/VehicleControl1/CreateBus VhclCtrl.Steering ==
  In1 : Inport
  Bus Creator : BusCreator  Inputs=5
  Demux : Demux  Outputs=5
  Out1 : Outport
  wires:
  In1/1 -> Demux/1
  Bus Creator/1 -> Out1/1
  Demux/1 -> Bus Creator/1  "VhclCtrl Steering Ang"
  Demux/5 -> Bus Creator/5  "VhclCtrl Steering ByTrq"
  Demux/3 -> Bus Creator/3  "VhclCtrl Steering AngAcc"
  Demux/2 -> Bus Creator/2  "VhclCtrl Steering AngVel"
  Demux/4 -> Bus Creator/4  "VhclCtrl Steering Trq"

== system TV2016_CAN/CarMaker/IPG Vehicle1/Brake/CreateBus Vhcl.Wheel.PT ==
  In : Inport
  BusCreator : BusCreator  Inputs=16
  Demux : Demux  Outputs=16
  Out : Outport
  wires:
  Demux/16 -> BusCreator/16  "Vhcl Wheel RR WhlBearing"
  Demux/15 -> BusCreator/15  "Vhcl Wheel RR Trq_T2W"
  Demux/14 -> BusCreator/14  "Vhcl Wheel RR Trq_BrakeReg_trg"
  Demux/13 -> BusCreator/13  "Vhcl Wheel RR Trq_Brake"
  Demux/12 -> BusCreator/12  "Vhcl Wheel RL WhlBearing"
  Demux/11 -> BusCreator/11  "Vhcl Wheel RL Trq_T2W"
  Demux/10 -> BusCreator/10  "Vhcl Wheel RL Trq_BrakeReg_trg"
  Demux/9 -> BusCreator/9  "Vhcl Wheel RL Trq_Brake"
  Demux/8 -> BusCreator/8  "Vhcl Wheel FR WhlBearing"
  Demux/7 -> BusCreator/7  "Vhcl Wheel FR Trq_T2W"
  Demux/6 -> BusCreator/6  "Vhcl Wheel FR Trq_BrakeReg_trg"
  Demux/5 -> BusCreator/5  "Vhcl Wheel FR Trq_Brake"
  Demux/4 -> BusCreator/4  "Vhcl Wheel FL WhlBearing"
  Demux/3 -> BusCreator/3  "Vhcl Wheel FL Trq_T2W"
  Demux/2 -> BusCreator/2  "Vhcl Wheel FL Trq_BrakeReg_trg"
  Demux/1 -> BusCreator/1  "Vhcl Wheel FL Trq_Brake"
  BusCreator/1 -> Out/1
  In/1 -> Demux/1

== system TV2016_CAN/CarMaker/IPG Vehicle1/CarAndTrailer/CarAndTrailerUpd ==
  Sync_In : Inport
  Vhcl.Steering : Inport  Port=2
  Vhcl.Motion : Inport  Port=3
  Vhcl.PoI : Inport  Port=4
  Vhcl.Wheel.FL : Inport  Port=5
  Vhcl.Wheel.FR : Inport  Port=6
  Vhcl.Wheel.RL : Inport  Port=7
  Vhcl.Wheel.RR : Inport  Port=8
  Car.Hitch.FrcTrq : Inport  Port=9
  Vhcl.Fr1A : Inport  Port=10
  CarAndTrailerUpd : S-Function  FunctionName=CM_Sfun  Parameters='CarAndTrUpd'
  CreateBus Brake.IF.In : Subsystem
  Sync_Out : Outport
  Brake.IF.In : Outport  Port=2
  wires:
  Vhcl.Fr1A/1 -> CarAndTrailerUpd/10  "user vehicle only"
  Vhcl.Steering/1 -> CarAndTrailerUpd/2
  Vhcl.Motion/1 -> CarAndTrailerUpd/3
  Vhcl.PoI/1 -> CarAndTrailerUpd/4
  Vhcl.Wheel.FL/1 -> CarAndTrailerUpd/5
  Vhcl.Wheel.FR/1 -> CarAndTrailerUpd/6
  Car.Hitch.FrcTrq/1 -> CarAndTrailerUpd/9
  Vhcl.Wheel.RR/1 -> CarAndTrailerUpd/8
  Vhcl.Wheel.RL/1 -> CarAndTrailerUpd/7
  CarAndTrailerUpd/2 -> CreateBus Brake.IF.In/1(In)
  CreateBus Brake.IF.In/1(Out) -> Brake.IF.In/1
  CarAndTrailerUpd/1 -> Sync_Out/1
  Sync_In/1 -> CarAndTrailerUpd/1

== system TV2016_CAN/CarMaker/IPG Vehicle1/CarAndTrailer/Forces ==
  Sync_In : Inport
  TireFL_In : Inport  Port=2
  TireFR_In : Inport  Port=3
  TireRL_In : Inport  Port=4
  TireRR_In : Inport  Port=5
  lSpring : Inport  Port=6
  vDamp : Inport  Port=7
  lStabi : Inport  Port=8
  lBuf : Inport  Port=9
  External Suspension Forces : Subsystem
  Tires : Subsystem
  Vehicle Forces : Subsystem
  Sync_Out : Outport
  Car.Virtual : Outport  Port=2
  Car.Aero : Outport  Port=3
  Car.Load : Outport  Port=4
  TireFL_Out : Outport  Port=5
  TireFR_Out : Outport  Port=6
  TireRL_Out : Outport  Port=7
  TireRR_Out : Outport  Port=8
  FSpring : Outport  Port=9
  FDamp : Outport  Port=10
  FStabi : Outport  Port=11
  FBuf : Outport  Port=12
  wires:
  External Suspension Forces/4(FBuf) -> FBuf/1
  lBuf/1 -> External Suspension Forces/5(lBuf)
  Tires/1(TireFL_Out) -> TireFL_Out/1
  Tires/4(TireRR_Out) -> TireRR_Out/1
  Tires/3(TireRL_Out) -> TireRL_Out/1
  Tires/2(TireFR_Out) -> TireFR_Out/1
  TireRR_In/1 -> Tires/4(TireRR_In)
  TireRL_In/1 -> Tires/3(TireRL_In)
  TireFR_In/1 -> Tires/2(TireFR_In)
  Sync_In/1 -> External Suspension Forces/1(Sync_In), Tires/5(Sync_In), Vehicle Forces/1(Sync_In)
  Vehicle Forces/1(Sync_Out) -> Sync_Out/1
  TireFL_In/1 -> Tires/1(TireFL_In)
  Vehicle Forces/2(Car.Virtual) -> Car.Virtual/1
  Vehicle Forces/3(Car.Aero) -> Car.Aero/1
  Vehicle Forces/4(Car.Load) -> Car.Load/1
  lSpring/1 -> External Suspension Forces/2(lSpring)
  External Suspension Forces/2(FDamp) -> FDamp/1
  vDamp/1 -> External Suspension Forces/3(vDamp)
  lStabi/1 -> External Suspension Forces/4(lStabi)
  External Suspension Forces/3(FStabi) -> FStabi/1
  External Suspension Forces/1(FSpring) -> FSpring/1

== system TV2016_CAN/CarMaker/IPG Vehicle1/CarAndTrailer/Kinematics ==
  Sync_In : Inport
  Steer.IF : Inport  Port=2
  Kinematics : S-Function  FunctionName=CM_Sfun  Parameters='Kinematics'
  Sync_Out : Outport
  TireFL_In : Outport  Port=2
  TireFR_In : Outport  Port=3
  TireRL_In : Outport  Port=4
  TireRR_In : Outport  Port=5
  lSpring : Outport  Port=6
  vDamp : Outport  Port=7
  lStabi : Outport  Port=8
  lBuf : Outport  Port=9
  wires:
  Kinematics/9 -> lBuf/1
  Kinematics/8 -> lStabi/1
  Kinematics/2 -> TireFL_In/1
  Kinematics/3 -> TireFR_In/1
  Kinematics/4 -> TireRL_In/1
  Kinematics/5 -> TireRR_In/1
  Kinematics/6 -> lSpring/1
  Kinematics/7 -> vDamp/1
  Sync_In/1 -> Kinematics/1
  Kinematics/1 -> Sync_Out/1
  Steer.IF/1 -> Kinematics/2

== system TV2016_CAN/CarMaker/IPG Vehicle1/CarAndTrailer/Kinetics ==
  Sync_In : Inport
  Car.Virtual : Inport  Port=2
  Car.Aero : Inport  Port=3
  Car.Load : Inport  Port=4
  TireFL.Out : Inport  Port=5
  TireFR.Out : Inport  Port=6
  TireRL.Out : Inport  Port=7
  TireRR.Out : Inport  Port=8
  FSpring : Inport  Port=9
  FDamp : Inport  Port=10
  FStabi : Inport  Port=11
  FBuf : Inport  Port=12
  Bus Creator : BusCreator
  Bus Creator1 : BusCreator  Inputs=12
  Bus Creator2 : BusCreator  Inputs=6
  Bus Creator3 : BusCreator  Inputs=6
  Bus Creator4 : BusCreator
  Demux : Demux  Outputs=12
  Demux1 : Demux  Outputs=6
  Demux2 : Demux  Outputs=6
  Demux3 : Demux
  Demux4 : Demux
  Kinetics : S-Function  FunctionName=CM_Sfun  Parameters='Kinetics'
  Sync_Out : Outport
  Trailer.Load : Outport  Port=2
  Car.Hitch : Outport  Port=3
  Car.Fr1 : Outport  Port=4
  Car.Trq_T2W : Outport  Port=5
  WheelCarrier.Misc : Outport  Port=6
  wires:
  FBuf/1 -> Kinetics/12
  Sync_In/1 -> Kinetics/1
  Kinetics/1 -> Sync_Out/1
  Car.Aero/1 -> Kinetics/3
  Car.Virtual/1 -> Kinetics/2
  Bus Creator1/1 -> Trailer.Load/1
  Demux/1 -> Bus Creator1/1  "Trailer Load_0 mass"
  Demux/2 -> Bus Creator1/2  "Trailer Load_0 tx"
  Demux/3 -> Bus Creator1/3  "Trailer Load_0 ty"
  Demux/4 -> Bus Creator1/4  "Trailer Load_0 tz"
  Kinetics/2 -> Demux/1
  Demux/5 -> Bus Creator1/5  "Trailer Load_1 mass"
  Demux/6 -> Bus Creator1/6  "Trailer Load_1 tx"
  Demux/7 -> Bus Creator1/7  "Trailer Load_1 ty"
  Demux/8 -> Bus Creator1/8  "Trailer Load_1 tz"
  Demux/9 -> Bus Creator1/9  "Trailer Load_2 mass"
  Demux/10 -> Bus Creator1/10  "Trailer Load_2 tx"
  Demux/11 -> Bus Creator1/11  "Trailer Load_2 ty"
  Demux/12 -> Bus Creator1/12  "Trailer Load_2 tz"
  Demux1/1 -> Bus Creator2/1  "Car Hitch tx"
  Demux1/2 -> Bus Creator2/2  "Car Hitch ty"
  Demux1/3 -> Bus Creator2/3  "Car Hitch tz"
  Demux1/4 -> Bus Creator2/4  "Car Hitch vx"
  Demux1/5 -> Bus Creator2/5  "Car Hitch vy"
  Demux1/6 -> Bus Creator2/6  "Car Hitch vz"
  Kinetics/3 -> Demux1/1
  Bus Creator2/1 -> Car.Hitch/1
  Demux2/1 -> Bus Creator3/1  "Car Fr1 rx"
  Demux2/2 -> Bus Creator3/2  "Car Fr1 ry"
  Demux2/3 -> Bus Creator3/3  "Car Fr1 rz"
  Demux2/4 -> Bus Creator3/4  "Car Fr1 rvx"
  Demux2/5 -> Bus Creator3/5  "Car Fr1 rvy"
  Demux2/6 -> Bus Creator3/6  "Car Fr1 rvz"
  Bus Creator3/1 -> Car.Fr1/1
  Kinetics/4 -> Demux2/1
  Car.Load/1 -> Kinetics/4
  Demux3/1 -> Bus Creator4/1  "car Susp FL GenInert2"
  Demux3/2 -> Bus Creator4/2  "car Susp FR GenInert2"
  Demux3/3 -> Bus Creator4/3  "car Susp FL GenFrc2"
  Demux3/4 -> Bus Creator4/4  "car Susp FR GenFrc2"
  Bus Creator4/1 -> WheelCarrier.Misc/1
  Bus Creator/1 -> Car.Trq_T2W/1
  Demux4/4 -> Bus Creator/4  "Car Trq_T2WRR"
  Demux4/3 -> Bus Creator/3  "Car Trq_T2WRL"
  Demux4/2 -> Bus Creator/2  "Car Trq_T2WFR"
  Demux4/1 -> Bus Creator/1  "Car Trq_T2WFL"
  TireFL.Out/1 -> Kinetics/5
  TireFR.Out/1 -> Kinetics/6
  TireRL.Out/1 -> Kinetics/7
  TireRR.Out/1 -> Kinetics/8
  FSpring/1 -> Kinetics/9
  FDamp/1 -> Kinetics/10
  FStabi/1 -> Kinetics/11
  Kinetics/6 -> Demux3/1
  Kinetics/5 -> Demux4/1

== system TV2016_CAN/CarMaker/IPG Vehicle1/CarAndTrailer/Steering ==
  note: When replacing the entire steering system,
      | be sure to add '-disablesteering' to the command line arguments
      | in the CarMaker Model Configuration block.
  Sync_In : Inport
  VhclCtrl.Steering : Inport  Port=2
  Bus Creator1 : BusCreator  Inputs=16
  Bus Creator2 : BusCreator
  Demux : Demux  Outputs=20
  Steering : S-Function  FunctionName=CM_Sfun  Parameters='Steering'
  Terminator : Terminator
  Sync_Out : Outport
  Steer.IF : Outport  Port=2
  wires:
  Bus Creator1/1 -> Steer.IF/1
  Steering/2 -> Demux/1
  Demux/8 -> Bus Creator1/8  "Steering IF AssistTrqPin"
  Demux/7 -> Bus Creator1/7  "Steering IF AssistTrqCol"
  Demux/6 -> Bus Creator1/6  "Steering IF AssistFrc"
  Demux/20 -> Bus Creator2/4  "Steering IF R Inert"
  Demux/17 -> Bus Creator2/1  "Steering IF L Frc"
  Demux/18 -> Bus Creator2/2  "Steering IF L Inert"
  Demux/19 -> Bus Creator2/3  "Steering IF R Frc"
  Bus Creator2/1 -> Terminator/1  "Steer IF (in)"
  Demux/16 -> Bus Creator1/16  "Steering IF R iSteer2q"
  Demux/9 -> Bus Creator1/9  "Steering IF L q"
  Demux/10 -> Bus Creator1/10  "Steering IF L qp"
  Demux/11 -> Bus Creator1/11  "Steering IF L qpp"
  Demux/12 -> Bus Creator1/12  "Steering IF L iSteer2q"
  Demux/13 -> Bus Creator1/13  "Steering IF R q"
  Demux/14 -> Bus Creator1/14  "Steering IF R qp"
  Demux/15 -> Bus Creator1/15  "Steering IF R qpp"
  VhclCtrl.Steering/1 -> Steering/2
  Steering/1 -> Sync_Out/1
  Sync_In/1 -> Steering/1
  Demux/1 -> Bus Creator1/1  "Steering IF Ang"
  Demux/2 -> Bus Creator1/2  "Steering IF AngVel"
  Demux/3 -> Bus Creator1/3  "Steering IF AngAcc"
  Demux/4 -> Bus Creator1/4  "Steering IF Trq"
  Demux/5 -> Bus Creator1/5  "Steering IF TrqStatic"

== system TV2016_CAN/CarMaker/IPG Vehicle1/CarAndTrailer/Trailer ==
  Sync_In : Inport
  Trailer.Load : Inport  Port=2
  Car.Hitch : Inport  Port=3
  Car.Fr1 : Inport  Port=4
  Car.Trq_T2W : Inport  Port=5
  WheelCarrier.Misc : Inport  Port=6
  CreateBus Car.Hitch.FrcTrq : Subsystem
  CreateBus Vhcl.Motion : Subsystem
  CreateBus Vhcl.PoI : Subsystem
  CreateBus Vhcl.Steering : Subsystem
  CreateBus Vhcl.Wheel.FL : Subsystem
  CreateBus Vhcl.Wheel.FR : Subsystem
  CreateBus Vhcl.Wheel.RL : Subsystem
  CreateBus Vhcl.Wheel.RR : Subsystem
  Trailer : S-Function  FunctionName=CM_Sfun  Parameters='Trailer'
  Sync_Out : Outport
  Vhcl.Steering : Outport  Port=2
  Vhcl.Motion : Outport  Port=3
  Vhcl.PoI : Outport  Port=4
  Vhcl.Wheel.FL : Outport  Port=5
  Vhcl.Wheel.FR : Outport  Port=6
  Vhcl.Wheel.RL : Outport  Port=7
  Vhcl.Wheel.RR : Outport  Port=8
  Car.Hitch.FrcTrq : Outport  Port=9
  wires:
  Trailer/2 -> CreateBus Vhcl.Steering/1(In1)
  CreateBus Vhcl.Steering/1(Out1) -> Vhcl.Steering/1
  Trailer/3 -> CreateBus Vhcl.Motion/1(In1)
  Trailer/4 -> CreateBus Vhcl.PoI/1(In1)
  Trailer/5 -> CreateBus Vhcl.Wheel.FL/1(In1)
  Trailer/6 -> CreateBus Vhcl.Wheel.FR/1(In1)
  Trailer/7 -> CreateBus Vhcl.Wheel.RL/1(In1)
  Trailer/9 -> CreateBus Car.Hitch.FrcTrq/1(In1)
  Trailer/8 -> CreateBus Vhcl.Wheel.RR/1(In1)
  CreateBus Vhcl.Wheel.RR/1(Out1) -> Vhcl.Wheel.RR/1  "Vhcl.Wheel.RR"
  CreateBus Vhcl.Wheel.RL/1(Out1) -> Vhcl.Wheel.RL/1  "Vhcl.Wheel.RL"
  CreateBus Vhcl.Wheel.FR/1(Out1) -> Vhcl.Wheel.FR/1  "Vhcl.Wheel.FR"
  CreateBus Vhcl.Wheel.FL/1(Out1) -> Vhcl.Wheel.FL/1  "Vhcl.Wheel.FL"
  CreateBus Vhcl.PoI/1(Out1) -> Vhcl.PoI/1
  CreateBus Vhcl.Motion/1(Out1) -> Vhcl.Motion/1
  Car.Trq_T2W/1 -> Trailer/5
  WheelCarrier.Misc/1 -> Trailer/6
  CreateBus Car.Hitch.FrcTrq/1(Car.Hitch.FrcTrq) -> Car.Hitch.FrcTrq/1
  Car.Fr1/1 -> Trailer/4
  Car.Hitch/1 -> Trailer/3
  Trailer.Load/1 -> Trailer/2
  Trailer/1 -> Sync_Out/1
  Sync_In/1 -> Trailer/1
